simulink model "PIDLQR"  (Simulink 7.9)
settings: Solver=ode45  SolverMode=SingleTasking  StartTime=0  StopTime=10  MaxStep=0.02  RelTol=1e-3  AbsTol=1e-6
libraries: simulink x2
Description:
  | Inverted Pendulum with Animation
  | 
  | The animation is created using MATLAB(R) Handle Graphics(R).  The animation block is a masked
  | S-function.  For more information, use the context menu to look under the Animation block's mask
  | and open the S-function for editing.
settings Model: Creator=The MathWorks Inc.  LastModifiedBy=SRH  ExtModeAutoUpdateStatusClock=off
settings DataIOCC: ExternalInput=[]  InitialState=[]  LimitDataPoints=off  SaveOutput=off  SaveTime=off
settings OptimizationCC: BlockReduction=off  BooleanDataType=off  InitFltsAndDblsToZero=on
settings DebuggingCC: SaveWithParameterizedLinksMsg=none  SignalResolutionControl=TryResolveAllWithWarning  SolverPrmCheckMsg=none  MultiTaskDSMMsg=warning  MultiTaskCondExecSysMsg=none  SigSpecEnsureSampleTimeMsg=none  FcnCallInpInsideContextMsg=Use local settings
settings HardwareCC: TargetUnknown=on
settings RTWCC: IncludeERTFirstTime=on
settings GRTTargetCC: TargetFcnLib=ansi_tfl_tmw.mat  CombineOutputUpdateFcns=off  GRTInterface=on

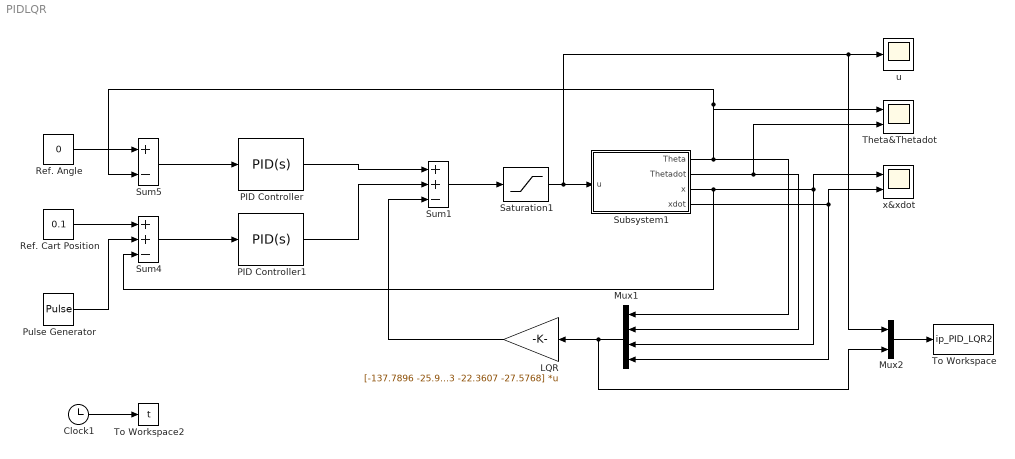
== system PIDLQR ==
  Clock1 : Clock
  LQR : Gain  Gain=[-137.7896 -25.9783 -22.3607 -27.5768]  Multiplication=Matrix(K*u)
  Mux1 : Mux
  Mux2 : Mux  Inputs=2
  PID Controller : simulink/Continuous/PID Controller  Controller=PID  TimeDomain=Continuous-time  SampleTime=1  IntegratorMethod=Forward Euler  FilterMethod=Forward Euler  Form=Parallel  P=1  I=1  D=1  N=100  InitialConditionSource=internal  InitialConditionForIntegrator=0  InitialConditionForFilter=0  ExternalReset=none  LimitOutput=off  UpperSaturationLimit=inf  LowerSaturationLimit=-inf  LinearizeAsGain=off  AntiWindupMode=none  Kb=1  TrackingMode=off  Kt=1  PParamMin=[]  PParamMax=[]  IParamMin=[]  IParamMax=[]  DParamMin=[]  DParamMax=[]  NParamMin=[]  NParamMax=[]  KbParamMin=[]  KbParamMax=[]  KtParamMin=[]  KtParamMax=[]  POutMin=[]  POutMax=[]  IOutMin=[]  IOutMax=[]  DOutMin=[]  DOutMax=[]  NOutMin=[]  NOutMax=[]  KbOutMin=[]  KbOutMax=[]  KtOutMin=[]  KtOutMax=[]  IntegratorOutMin=[]  IntegratorOutMax=[]  FilterOutMin=[]  FilterOutMax=[]  SumOutMin=[]  SumOutMax=[]  SumI1OutMin=[]  SumI1OutMax=[]  SumI2OutMin=[]  SumI2OutMax=[]  SumI3OutMin=[]  SumI3OutMax=[]  SumDOutMin=[]  SumDOutMax=[]  SaturationOutMin=[]  SaturationOutMax=[]  IntegratorContinuousStateAttributes=''  IntegratorStateMustResolveToSignalObject=off  IntegratorRTWStateStorageClass=Auto  FilterContinuousStateAttributes=''  FilterStateMustResolveToSignalObject=off  FilterRTWStateStorageClass=Auto
  PID Controller1 : simulink/Continuous/PID Controller  Controller=PID  TimeDomain=Continuous-time  SampleTime=1  IntegratorMethod=Forward Euler  FilterMethod=Forward Euler  Form=Parallel  P=1.5  I=-7.5  D=5  N=100  InitialConditionSource=internal  InitialConditionForIntegrator=0  InitialConditionForFilter=0  ExternalReset=none  LimitOutput=off  UpperSaturationLimit=inf  LowerSaturationLimit=-inf  LinearizeAsGain=off  AntiWindupMode=none  Kb=1  TrackingMode=off  Kt=1  PParamMin=[]  PParamMax=[]  IParamMin=[]  IParamMax=[]  DParamMin=[]  DParamMax=[]  NParamMin=[]  NParamMax=[]  KbParamMin=[]  KbParamMax=[]  KtParamMin=[]  KtParamMax=[]  POutMin=[]  POutMax=[]  IOutMin=[]  IOutMax=[]  DOutMin=[]  DOutMax=[]  NOutMin=[]  NOutMax=[]  KbOutMin=[]  KbOutMax=[]  KtOutMin=[]  KtOutMax=[]  IntegratorOutMin=[]  IntegratorOutMax=[]  FilterOutMin=[]  FilterOutMax=[]  SumOutMin=[]  SumOutMax=[]  SumI1OutMin=[]  SumI1OutMax=[]  SumI2OutMin=[]  SumI2OutMax=[]  SumI3OutMin=[]  SumI3OutMax=[]  SumDOutMin=[]  SumDOutMax=[]  SaturationOutMin=[]  SaturationOutMax=[]  IntegratorContinuousStateAttributes=''  IntegratorStateMustResolveToSignalObject=off  IntegratorRTWStateStorageClass=Auto  FilterContinuousStateAttributes=''  FilterStateMustResolveToSignalObject=off  FilterRTWStateStorageClass=Auto
  Pulse Generator : DiscretePulseGenerator  PulseType=Time based  Amplitude=0  Period=10  PulseWidth=5
  Ref. Angle : Constant  Value=0
  Ref. Cart Position : Constant  Value=0.1
  Saturation1 : Saturate  UpperLimit=100  LowerLimit=-100
  Subsystem1 : Subsystem
  Sum1 : Sum  Inputs=++-  SaturateOnIntegerOverflow=on  InputSameDT=on  OutDataTypeStr=Inherit: Same as first input
  Sum4 : Sum  Inputs=++-  SaturateOnIntegerOverflow=on  InputSameDT=on  OutDataTypeStr=Inherit: Same as first input
  Sum5 : Sum  Inputs=+-  SaturateOnIntegerOverflow=on  InputSameDT=on  OutDataTypeStr=Inherit: Same as first input
  Theta&Thetadot : Scope  NumInputPorts=2
      settings: YMin=-5~-5  YMax=5~5
  To Workspace : ToWorkspace  VariableName=ip_PID_LQR2  SampleTime=-1
  To Workspace2 : ToWorkspace  VariableName=t  SampleTime=-1
  u : Scope
  x&xdot : Scope  NumInputPorts=2
      settings: YMin=-5~-5  YMax=5~5  SaveName=ScopeData4
  wires:
  Subsystem1/1(Theta) -> Mux1/1, Sum5/2, Theta&Thetadot/1
  Subsystem1/2(Thetadot) -> Mux1/2, Theta&Thetadot/2
  Subsystem1/3(x) -> Sum4/3, Mux1/3, x&xdot/1
  Subsystem1/4(xdot) -> Mux1/4, x&xdot/2
  Mux1/1 -> LQR/1, Mux2/2
  Sum1/1 -> Saturation1/1
  Saturation1/1 -> Subsystem1/1(u), u/1, Mux2/1
  LQR/1 -> Sum1/3
  Sum4/1 -> PID Controller1/1
  Sum5/1 -> PID Controller/1
  PID Controller/1 -> Sum1/1
  PID Controller1/1 -> Sum1/2
  Ref. Angle/1 -> Sum5/1
  Ref. Cart Position/1 -> Sum4/1
  Pulse Generator/1 -> Sum4/2
  Clock1/1 -> To Workspace2/1
  Mux2/1 -> To Workspace/1

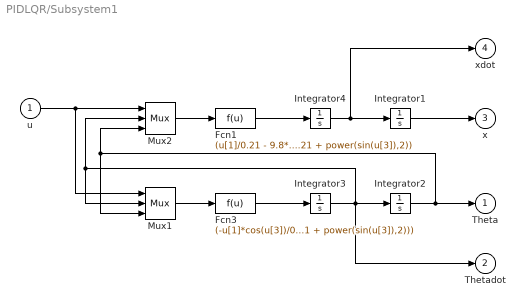
== system PIDLQR/Subsystem1 ==
  u : Inport
  Fcn1 : Fcn  Expr=(u[1]/0.21 - 9.8*sin(u[3])*cos(u[3]) + (0.61/2)*power(u[2],2)*sin(u[3]))/(0.455/0.21 + power(sin(u[3]),2))
  Fcn3 : Fcn  Expr=(-u[1]*cos(u[3])/0.21 + (0.455+0.21)*9.8*sin(u[3])/0.21 - (0.61/2)*power(u[2],2)*sin(u[3])*cos(u[3]))/((0.61/2)*(0.455/0.21 + power(sin(u[3]),2)))
  Integrator{1..4} (4 alike) : Integrator
  Mux1 : Mux  Inputs=3
  Mux2 : Mux  Inputs=3
  Theta : Outport  InitialOutput=0
  Thetadot : Outport  Port=2  InitialOutput=0
  x : Outport  Port=3  InitialOutput=0
  xdot : Outport  Port=4  InitialOutput=0
  wires:
  Integrator1/1 -> x/1
  Fcn3/1 -> Integrator3/1
  Mux1/1 -> Fcn3/1
  Mux2/1 -> Fcn1/1
  Fcn1/1 -> Integrator4/1
  Integrator4/1 -> Integrator1/1, xdot/1
  u/1 -> Mux2/1, Mux1/1
  Integrator3/1 -> Integrator2/1, Mux2/2, Mux1/2, Thetadot/1
  Integrator2/1 -> Theta/1, Mux2/3, Mux1/3
